simulink model "Final_Project"  (R2019a)
settings: Solver=VariableStepAuto  StartTime=0.0  StopTime=100.0  RelTol=1e-3
undefined symbols (not defined in the file): sigbuilder_block
libraries: nesl_utility x42, fl_lib x33, sh_lib x28
settings Model: Creator=danis  LastModifiedBy=danis

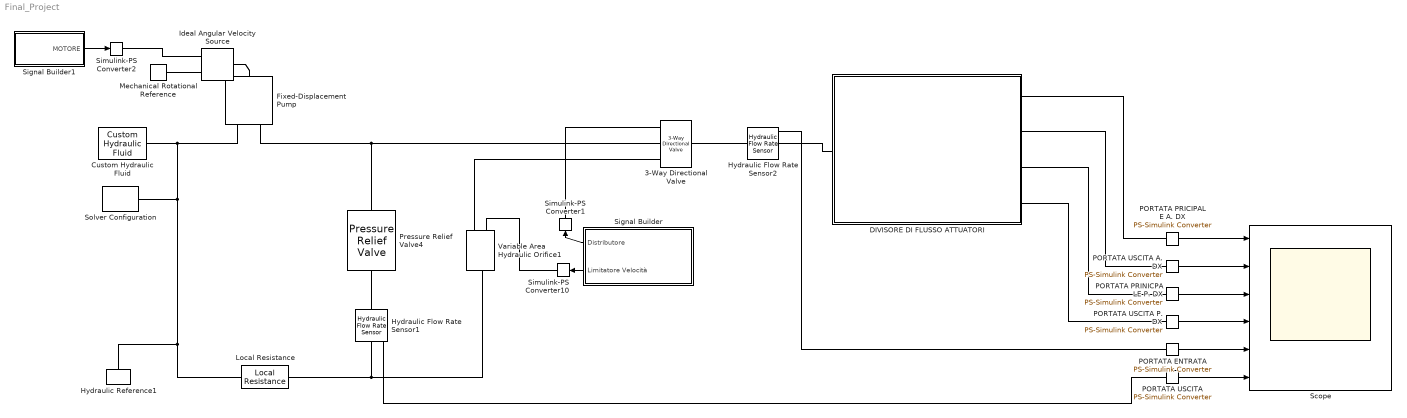
== system Final_Project ==
  3-Way Directional Valve : sh_lib/Valves/Directional Valves/3-Way Directional Valve  area_spec=sh.valves.directional_valves.enum.area_spec.identical  x_0_P=0 m  x_0_T=0 m  mdl_type_identical=sh.valves.directional_valves.enum.mdl_type.linear  mdl_type_different=sh.valves.directional_valves.enum.mdl_type.linear  opening_max=0.005 m  area_max=0.5e-4 m^2  opening_max_P_A=0.005 m  area_max_P_A=0.5e-4 m^2  opening_max_A_T=0.005 m  area_max_A_T=0.5e-4 m^2  opening_area_tab=[-.002, 0, .002, .005, .015] m  area_tab=[1e-09, 2.0352e-07, 4.0736e-05, .00011438, .00034356] m^2  opening_flow_rate_tab=[-.002, 0, .002, .005, .015] m  pressure_tab=[-10000000, -5000000, -2000000, 2000000, 5000000, 10000000] Pa  flow_rate_tab=[-1e-07, -7.0711e-08, -4.4721e-08, 4.4721e-08, 7.0711e-08, 1e-07; -2.0352e-05, -1.4391e-05, -9.1017e-06, 9.1017e-06, 1.4391e-05, 2.0352e-05; -.0040736, -.0028805, -.0018218, .0018218, .0028805, .0040736; -.011438, -.0080879, -.0051152, .0051152, .0080879, .011438; -.034356, -.024293, -.015364, .015364, .024293, .034356] m^3/s  opening_area_tab_P_A=[-.002, 0, .002, .005, .015] m  area_tab_P_A=[1e-09, 2.0352e-07, 4.0736e-05, .00011438, .00034356] m^2  opening_flow_rate_tab_P_A=[-.002, 0, .002, .005, .015] m  pressure_tab_P_A=[-10000000, -5000000, -2000000, 2000000, 5000000, 10000000] Pa  flow_rate_tab_P_A=[-1e-07, -7.0711e-08, -4.4721e-08, 4.4721e-08, 7.0711e-08, 1e-07; -2.0352e-05, -1.4391e-05, -9.1017e-06, 9.1017e-06, 1.4391e-05, 2.0352e-05; -.0040736, -.0028805, -.0018218, .0018218, .0028805, .0040736; -.011438, -.0080879, -.0051152, .0051152, .0080879, .011438; -.034356, -.024293, -.015364, .015364, .024293, .034356] m^3/s  opening_area_tab_A_T=[-.002, 0, .002, .005, .015] m  area_tab_A_T=[1e-09, 2.0352e-07, 4.0736e-05, .00011438, .00034356] m^2  opening_flow_rate_tab_A_T=[-.002, 0, .002, .005, .015] m  pressure_tab_A_T=[-10000000, -5000000, -2000000, 2000000, 5000000, 10000000] Pa  flow_rate_tab_A_T=[-1e-07, -7.0711e-08, -4.4721e-08, 4.4721e-08, 7.0711e-08, 1e-07; -2.0352e-05, -1.4391e-05, -9.1017e-06, 9.1017e-06, 1.4391e-05, 2.0352e-05; -.0040736, -.0028805, -.0018218, .0018218, .0028805, .0040736; -.011438, -.0080879, -.0051152, .0051152, .0080879, .011438; -.034356, -.024293, -.015364, .015364, .024293, .034356] m^3/s  interp_method_identical=sh.valves.directional_valves.enum.interp_method.linear  interp_method_different=sh.valves.directional_valves.enum.interp_method.linear  extrap_method_identical=sh.valves.directional_valves.enum.extrap_method.linear  extrap_method_different=sh.valves.directional_valves.enum.extrap_method.linear  A_leak=1e-15 m^2  C_d=0.7  lam_spec=sh.valves.directional_valves.enum.lam_spec.pressure_ratio  B_lam=0.999  Re_cr=12
      settings: SourceProductName=Simscape Fluids  SourceProductBaseCode=SH
  Custom Hydraulic Fluid : fl_lib/Hydraulic/Hydraulic Utilities/Custom Hydraulic Fluid  density=870 kg/m^3  viscosity_kin=0.000046 m^2/s  bulk=0.8e9 Pa  alpha=0.005  range_error=2
      settings: SourceProductName=Foundation Library
  DIVISORE DI FLUSSO ATTUATORI : Subsystem
  Fixed-Displacement Pump : sh_lib/Pumps and Motors/Fixed-Displacement Pump  D=10.5 cm^3/rev  loss_spec=1  w_nominal=952.4 rpm  pr_nominal=100e7 Pa  visc_nominal=0.000046 m^2/s  dens_nominal=870 kg/m^3  efficiency_vol=0.95  no_load_torque=0.0005 N*m  torque_pressure_coeff=0.6e-8 N*m/Pa  p_diff_eff_TLU=[100000, 1000000, 2000000] Pa  omega_eff_TLU=[25, 50, 100, 200, 300, 400] rad/s  vol_eff_TLU=[.816, .908, .954, .977, .981, .984; .325, .663, .831, .916, .925, .946; .137, .568, .78, .892, .893, .91]  mech_eff_TLU=[.996, .996, .996, .996, .996, .996; .988, .989, .989, .989, .989, .99; .981, .981, .982, .982, .983, .984]  p_diff_loss_TLU=[100000, 1000000, 2000000] Pa  omega_loss_TLU=[25, 50, 100, 200, 300, 400] rad/s  vol_loss_TLU=[.023, .023, .023, .023, .0285, .032; .0844, .0842, .0845, .084, .1125, .108; .1079, .108, .11, .108, .1605, .18] * 1e-3 m^3/s  mech_loss_TLU=[.002, .002, .002, .002, .002, .002; .0607, .0556, .0556, .0556, .0556, .0505; .1937, .1937, .1833, .1833, .1729, .1626] N*m  pressure_threshold=1e5 Pa  omega_threshold=10 rad/s  quadrant_check=0  pressure_check=0  min_valid_pressure=0 Pa  vol_eff_min=1e-3  vol_eff_max=1  mech_eff_min=1e-3  mech_eff_max=1
      settings: SourceProductName=Simscape Fluids  SourceProductBaseCode=SH
  Hydraulic Flow Rate Sensor1 : fl_lib/Hydraulic/Hydraulic Sensors/Hydraulic Flow Rate Sensor
      settings: SourceProductName=Simscape
  Hydraulic Flow Rate Sensor2 : fl_lib/Hydraulic/Hydraulic Sensors/Hydraulic Flow Rate Sensor
      settings: SourceProductName=Simscape
  Hydraulic Reference1 : fl_lib/Hydraulic/Hydraulic Elements/Hydraulic Reference
      settings: SourceProductName=Foundation Library
  Ideal Angular Velocity Source : fl_lib/Mechanical/Mechanical Sources/Ideal Angular Velocity Source
  Local Resistance : sh_lib/Local Hydraulic Resistances/Local Resistance  area=1e-4 m^2  mdl_type=1  kp_d=2  kp_r=2  lam_spec=1  B_lam=0.999  Re_cr=150  Re_vec=[-4000, -3000, -2000, -1000, -500, -200, -100, -50, -40, -30, -20, -15, -10, 10, 20, 30, 40, 50, 100, 200, 500, 1000, 2000, 4000, 5000, 10000]  loss_coeff_vec=[.25, .3, .65, .9, .65, .75, .9, 1.15, 1.35, 1.65, 2.3, 2.8, 3.1, 5, 2.7, 1.8, 1.46, 1.3, .9, .65, .42, .3, .2, .4, .42, .25]  interp_method=2  extrap_method=2  flow_rate_threshold=1e-6 m^3/s  flow_rate_specify=off  flow_rate_priority=None  flow_rate=0 m^3/s  flow_rate_nominal_specify=off  flow_rate_nominal_unit=m^3/s  flow_rate_nominal_value=1  pressure_drop_specify=off  pressure_drop_priority=None  pressure_drop=0 Pa  pressure_drop_nominal_specify=off  pressure_drop_nominal_unit=Pa  pressure_drop_nominal_value=1
      settings: SourceProductName=Simscape Fluids  SourceProductBaseCode=SH
  Mechanical Rotational Reference : fl_lib/Mechanical/Rotational Elements/Mechanical Rotational Reference
  PORTATA ENTRATA : nesl_utility/PS-Simulink Converter  PhysicalDomain=network_engine_domain  SubClassName=ps_output  LeftPortType=input  RightPortType=output  PseudoPeriodic=off  Frequencies=[]  Unit=1  AffineConversion=off
  PORTATA PRICIPALE A. DX : nesl_utility/PS-Simulink Converter  PhysicalDomain=network_engine_domain  SubClassName=ps_output  LeftPortType=input  RightPortType=output  PseudoPeriodic=off  Frequencies=[]  Unit=1  AffineConversion=off
  PORTATA PRINICPALE P. DX : nesl_utility/PS-Simulink Converter  PhysicalDomain=network_engine_domain  SubClassName=ps_output  LeftPortType=input  RightPortType=output  PseudoPeriodic=off  Frequencies=[]  Unit=1  AffineConversion=off
  "PORTATA USCITA " : nesl_utility/PS-Simulink Converter  PhysicalDomain=network_engine_domain  SubClassName=ps_output  LeftPortType=input  RightPortType=output  PseudoPeriodic=off  Frequencies=[]  Unit=1  AffineConversion=off
  PORTATA USCITA A. DX : nesl_utility/PS-Simulink Converter  PhysicalDomain=network_engine_domain  SubClassName=ps_output  LeftPortType=input  RightPortType=output  PseudoPeriodic=off  Frequencies=[]  Unit=1  AffineConversion=off
  PORTATA USCITA P. DX : nesl_utility/PS-Simulink Converter  PhysicalDomain=network_engine_domain  SubClassName=ps_output  LeftPortType=input  RightPortType=output  PseudoPeriodic=off  Frequencies=[]  Unit=1  AffineConversion=off
  Pressure Relief Valve4 : sh_lib/Valves/Pressure Control Valves/Pressure Relief Valve  valve_area_spec=1  p_diff_TLU=[30.15e5 : 15e3 : 31.35e5] Pa  area_TLU=[1 : 1 : 9] .* 1e-5 m^2  area_max=1e-4 m^2  pres_set=75 bar  reg_range=5 bar  C_d=0.7  A_leak=1e-15 m^2  lam_spec=1  B_lam=0.999  Re_cr=12  dynamic=0  tau=0.1 s  area_init=1e-12 m^2
      settings: SourceProductName=Simscape Fluids  SourceProductBaseCode=SH
  Scope : Scope  NumInputPorts=6
  Signal Builder : Subsystem  Tag=STV Subsys  LoadFcn=sigbuilder_block('load');  StartFcn=sigbuilder_block('start');  StopFcn=sigbuilder_block('stop');  ClipboardFcn=sigbuilder_block('clipboard');  mask(Sigbuilder block){tuvar=[0:10]}
      mask help: Simulink:masks:SigbuilderBlock_MD
      mask init:
      | if ~strcmp(get_param(bdroot(gcbh),'SimulationStatus'),'stopped') tuvar = sigbuilder_block('maskInit'); end
      settings: CopyFcn=sigbuilder_block('copy');  DeleteFcn=sigbuilder_block('delete');  ModelCloseFcn=sigbuilder_block('modelClose');  PreSaveFcn=sigbuilder_block('preSave');  PauseFcn=sigbuilder_block('pause');  ContinueFcn=sigbuilder_block('continue');  NameChangeFcn=sigbuilder_block('namechange');  OpenFcn=sigbuilder_block('open',[154.868 35.3208 673.811 360.679 ]);  CloseFcn=sigbuilder_block('close');
      mask Display: plot(0, 0, 100, 100,[2, 2, 32, 32, 2], [68, 8, 8, 68, 68],[32, 2], [38, 38], [32, 19, 2],[53, 60, 44], [32, 17, 17, 2],[16, 16, 31, 31]);txt = getActiveGroup(gcbh);text(2, 100, txt,'verticalAlignment', 'top');
  Signal Builder1 : Subsystem  Tag=STV Subsys  LoadFcn=sigbuilder_block('load');  StartFcn=sigbuilder_block('start');  StopFcn=sigbuilder_block('stop');  ClipboardFcn=sigbuilder_block('clipboard');  mask(Sigbuilder block){tuvar=[0:10]}
      mask help: Simulink:masks:SigbuilderBlock_MD
      mask init:
      | if ~strcmp(get_param(bdroot(gcbh),'SimulationStatus'),'stopped') tuvar = sigbuilder_block('maskInit'); end
      settings: CopyFcn=sigbuilder_block('copy');  DeleteFcn=sigbuilder_block('delete');  ModelCloseFcn=sigbuilder_block('modelClose');  PreSaveFcn=sigbuilder_block('preSave');  PauseFcn=sigbuilder_block('pause');  ContinueFcn=sigbuilder_block('continue');  NameChangeFcn=sigbuilder_block('namechange');  OpenFcn=sigbuilder_block('open',[371.547 99.1698 550.868 360.679 ]);  CloseFcn=sigbuilder_block('close');
      mask Display: plot(0, 0, 100, 100,[2, 2, 32, 32, 2], [68, 8, 8, 68, 68],[32, 2], [38, 38], [32, 19, 2],[53, 60, 44], [32, 17, 17, 2],[16, 16, 31, 31]);txt = getActiveGroup(gcbh);text(2, 100, txt,'verticalAlignment', 'top');
  Simulink-PS Converter1 : nesl_utility/Simulink-PS Converter  PhysicalDomain=network_engine_domain  SubClassName=ps_input  LeftPortType=input  RightPortType=output  PseudoPeriodic=off  Frequencies=[]  NoiseDistribution=none  NoiseParameters=[]  Unit=1  AffineConversion=off  FilteringAndDerivatives=provide  SimscapeFilterOrder=1  InputFilterTimeConstant=0.001  UdotUserProvided=0
  Simulink-PS Converter10 : nesl_utility/Simulink-PS Converter  PhysicalDomain=network_engine_domain  SubClassName=ps_input  LeftPortType=input  RightPortType=output  PseudoPeriodic=off  Frequencies=[]  NoiseDistribution=none  NoiseParameters=[]  Unit=1  AffineConversion=off  FilteringAndDerivatives=provide  SimscapeFilterOrder=1  InputFilterTimeConstant=0.001  UdotUserProvided=0
  Simulink-PS Converter2 : nesl_utility/Simulink-PS Converter  PhysicalDomain=network_engine_domain  SubClassName=ps_input  LeftPortType=input  RightPortType=output  PseudoPeriodic=off  Frequencies=[]  NoiseDistribution=none  NoiseParameters=[]  Unit=1  AffineConversion=off  FilteringAndDerivatives=provide  SimscapeFilterOrder=1  InputFilterTimeConstant=0.001  UdotUserProvided=0
  Solver Configuration : nesl_utility/Solver Configuration  PhysicalDomain=network_engine_domain  SubClassName=solver  LeftPortType=input  RightPortType=generic  Tones=[]  Harmonics=[]  SimulateNoise=off  Profile=off  UseLocalSampling=off  EnableSwitchedLinearOptims=on  FrequencyDomain=off  UseCCode=off  RelTol=0.001  AbsTol=1e-06  MinStep=1e-09  ToWorkspace=off  RevertToSquareIcSolve=off  NumHomotopyIterations=100  PhasorMode=off  PhasorModeNumHarmonics=1  DoDC=off  ResidualTolerance=1e-09  UseLocalSolver=off  LocalSolverChoice=NE_BACKWARD_EULER_ADVANCER  LocalSolverSampleTime=0.001  DoFixedCost=off  MaxNonlinIter=3  MaxModeIter=2  LinearAlgebra=auto  EquationFormulation=NE_TIME_EF  DelaysMemoryBudget=1024  AutomaticFiltering=on  FilteringTimeConstant=0.001  PartitionStorageMethod=AS_NEEDED  PartitionMemoryBudget=1024  PartitionMethod=FAST
  Variable Area Hydraulic Orifice1 : fl_lib/Hydraulic/Hydraulic Elements/Variable Area Hydraulic Orifice  C_d=0.7  min_area=1e-12 m^2  lam_spec=1  B_lam=0.999  Re_cr=12  q_specify=off  q_priority=None  q=0.001 m^3/s  q_nominal_specify=off  q_nominal_unit=m^3/s  q_nominal_value=1  p_specify=off  p_priority=None  p=0 Pa  p_nominal_specify=off  p_nominal_unit=Pa  p_nominal_value=1
      settings: SourceProductName=Simscape  SourceProductBaseCode=SS
  wires:
  Signal Builder/1(Distributore) -> Simulink-PS Converter1/1
  Signal Builder/2(Limitatore Velocità) -> Simulink-PS Converter10/1
  PORTATA PRICIPALE A. DX/1 -> Scope/1
  PORTATA USCITA A. DX/1 -> Scope/2
  PORTATA PRINICPALE P. DX/1 -> Scope/3
  PORTATA USCITA P. DX/1 -> Scope/4
  PORTATA ENTRATA/1 -> Scope/5
  "PORTATA USCITA "/1 -> Scope/6
  Signal Builder1/1(MOTORE) -> Simulink-PS Converter2/1
  connections:
  3-Way Directional Valve/RConn3 -- Variable Area Hydraulic Orifice1/LConn2
  Simulink-PS Converter10/RConn1 -- Variable Area Hydraulic Orifice1/LConn1
  Simulink-PS Converter1/RConn1 -- 3-Way Directional Valve/RConn1
  Hydraulic Flow Rate Sensor1/LConn1 -- Pressure Relief Valve4/RConn1
  Hydraulic Flow Rate Sensor2/RConn2 -- DIVISORE DI FLUSSO ATTUATORI/LConn1
  Hydraulic Reference1/LConn1 -- Fixed-Displacement Pump/RConn2 -- Custom Hydraulic Fluid/RConn1 -- Solver Configuration/RConn1 -- Local Resistance/RConn1
  Variable Area Hydraulic Orifice1/RConn1 -- Local Resistance/LConn1 -- Hydraulic Flow Rate Sensor1/RConn2
  3-Way Directional Valve/LConn1 -- Hydraulic Flow Rate Sensor2/LConn1
  DIVISORE DI FLUSSO ATTUATORI/RConn1 -- PORTATA PRICIPALE A. DX/LConn1
  DIVISORE DI FLUSSO ATTUATORI/RConn2 -- PORTATA USCITA A. DX/LConn1
  DIVISORE DI FLUSSO ATTUATORI/RConn3 -- PORTATA PRINICPALE P. DX/LConn1
  DIVISORE DI FLUSSO ATTUATORI/RConn4 -- PORTATA USCITA P. DX/LConn1
  Hydraulic Flow Rate Sensor2/RConn1 -- PORTATA ENTRATA/LConn1
  Hydraulic Flow Rate Sensor1/RConn1 -- "PORTATA USCITA "/LConn1
  Ideal Angular Velocity Source/LConn1 -- Fixed-Displacement Pump/LConn1
  Ideal Angular Velocity Source/RConn2 -- Mechanical Rotational Reference/LConn1
  Simulink-PS Converter2/RConn1 -- Ideal Angular Velocity Source/RConn1
  3-Way Directional Valve/RConn2 -- Fixed-Displacement Pump/RConn1 -- Pressure Relief Valve4/LConn1

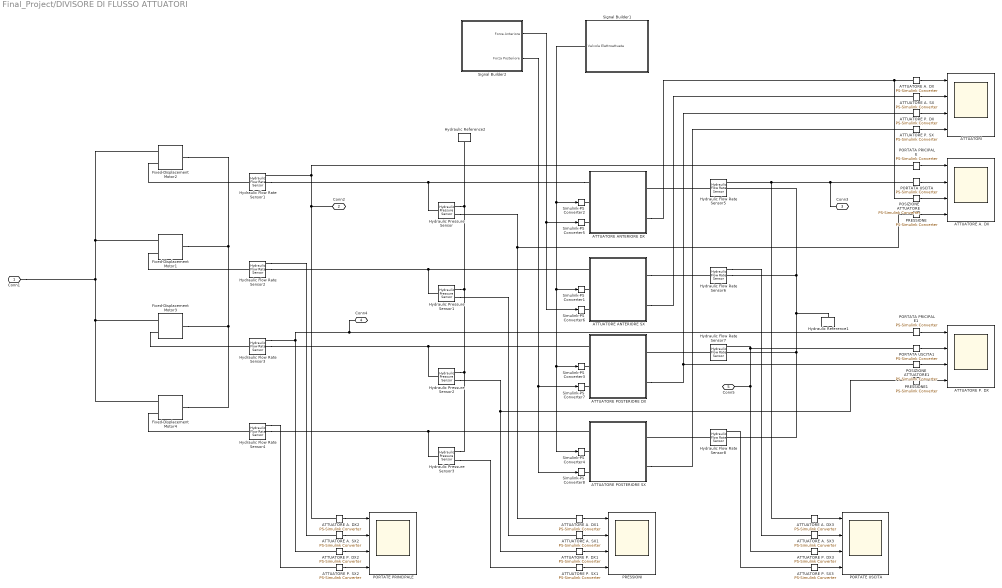
== system Final_Project/DIVISORE DI FLUSSO ATTUATORI ==
  ATTUATORE A. DX{,1..3} (4 alike) : nesl_utility/PS-Simulink Converter  PhysicalDomain=network_engine_domain  SubClassName=ps_output  LeftPortType=input  RightPortType=output  PseudoPeriodic=off  Frequencies=[]  Unit=1  AffineConversion=off
  "ATTUATORE A. DX " : Scope  NumInputPorts=4
  ATTUATORE A. SX{,1..3} (4 alike) : nesl_utility/PS-Simulink Converter  PhysicalDomain=network_engine_domain  SubClassName=ps_output  LeftPortType=input  RightPortType=output  PseudoPeriodic=off  Frequencies=[]  Unit=1  AffineConversion=off
  ATTUATORE ANTERIORE DX : Subsystem
  ATTUATORE ANTERIORE SX : Subsystem
  ATTUATORE P. DX{,1..3} (4 alike) : nesl_utility/PS-Simulink Converter  PhysicalDomain=network_engine_domain  SubClassName=ps_output  LeftPortType=input  RightPortType=output  PseudoPeriodic=off  Frequencies=[]  Unit=1  AffineConversion=off
  "ATTUATORE P. DX " : Scope  NumInputPorts=4
  ATTUATORE P. SX{,1..3} (4 alike) : nesl_utility/PS-Simulink Converter  PhysicalDomain=network_engine_domain  SubClassName=ps_output  LeftPortType=input  RightPortType=output  PseudoPeriodic=off  Frequencies=[]  Unit=1  AffineConversion=off
  ATTUATORE POSTERIORE DX : Subsystem
  ATTUATORE POSTERIORE SX : Subsystem
  ATTUATORI : Scope  NumInputPorts=4
  Fixed-Displacement Motor{1..4} (4 alike) : sh_lib/Pumps and Motors/Fixed-Displacement Motor  D=0.9 cm^3/rev  loss_spec=1  w_nominal=2777.8 rpm  pr_nominal=100e7 Pa  visc_nominal=0.000046 m^2/s  dens_nominal=870 kg/m^3  efficiency_vol=0.95  no_load_torque=0.0005 N*m  torque_pressure_coeff=0.6e-8 N*m/Pa  p_diff_eff_TLU=[100000, 1000000, 2000000] Pa  omega_eff_TLU=[25, 50, 100, 200, 300, 400] rad/s  vol_eff_TLU=[.816, .908, .954, .977, .981, .984; .325, .663, .831, .916, .925, .946; .137, .568, .78, .892, .893, .91]  mech_eff_TLU=[.996, .996, .996, .996, .996, .996; .988, .989, .989, .989, .989, .99; .981, .981, .982, .982, .983, .984]  p_diff_loss_TLU=[100000, 1000000, 2000000] Pa  omega_loss_TLU=[25, 50, 100, 200, 300, 400] rad/s  vol_loss_TLU=[.0282, .0253, .0241, .0235, .0291, .0325; .2596, .1271, .1017, .0917, .1216, .1142; .7874, .1901, .141, .1211, .1797, .1978] * 1e-3 m^3/s  mech_loss_TLU=[.002, .002, .002, .002, .002, .002; .06, .055, .055, .055, .055, .05; .19, .19, .18, .18, .17, .16] N*m  pressure_threshold=1e5 Pa  omega_threshold=10 rad/s  quadrant_check=0  pressure_check=0  min_valid_pressure=0 Pa  vol_eff_min=1e-3  vol_eff_max=1  mech_eff_min=1e-3  mech_eff_max=1
      settings: SourceProductName=Simscape Fluids  SourceProductBaseCode=SH
  Hydraulic Flow Rate Sensor{1..8} (8 alike) : fl_lib/Hydraulic/Hydraulic Sensors/Hydraulic Flow Rate Sensor
      settings: SourceProductName=Simscape
  Hydraulic Pressure Sensor{,1..3} (4 alike) : fl_lib/Hydraulic/Hydraulic Sensors/Hydraulic Pressure Sensor
      settings: SourceProductName=Simscape
  Hydraulic Reference1 : fl_lib/Hydraulic/Hydraulic Elements/Hydraulic Reference
      settings: SourceProductName=Foundation Library
  Hydraulic Reference2 : fl_lib/Hydraulic/Hydraulic Elements/Hydraulic Reference
      settings: SourceProductName=Foundation Library
  PORTATA PRICIPALE : nesl_utility/PS-Simulink Converter  PhysicalDomain=network_engine_domain  SubClassName=ps_output  LeftPortType=input  RightPortType=output  PseudoPeriodic=off  Frequencies=[]  Unit=1  AffineConversion=off
  PORTATA PRICIPALE1 : nesl_utility/PS-Simulink Converter  PhysicalDomain=network_engine_domain  SubClassName=ps_output  LeftPortType=input  RightPortType=output  PseudoPeriodic=off  Frequencies=[]  Unit=1  AffineConversion=off
  PORTATA USCITA : nesl_utility/PS-Simulink Converter  PhysicalDomain=network_engine_domain  SubClassName=ps_output  LeftPortType=input  RightPortType=output  PseudoPeriodic=off  Frequencies=[]  Unit=1  AffineConversion=off
  PORTATA USCITA1 : nesl_utility/PS-Simulink Converter  PhysicalDomain=network_engine_domain  SubClassName=ps_output  LeftPortType=input  RightPortType=output  PseudoPeriodic=off  Frequencies=[]  Unit=1  AffineConversion=off
  PORTATE PRINCIPALE : Scope  NumInputPorts=4
  PORTATE USCITA : Scope  NumInputPorts=4
  POSIZIONE ATTUATORE : nesl_utility/PS-Simulink Converter  PhysicalDomain=network_engine_domain  SubClassName=ps_output  LeftPortType=input  RightPortType=output  PseudoPeriodic=off  Frequencies=[]  Unit=1  AffineConversion=off
  POSIZIONE ATTUATORE1 : nesl_utility/PS-Simulink Converter  PhysicalDomain=network_engine_domain  SubClassName=ps_output  LeftPortType=input  RightPortType=output  PseudoPeriodic=off  Frequencies=[]  Unit=1  AffineConversion=off
  PRESSIONE : nesl_utility/PS-Simulink Converter  PhysicalDomain=network_engine_domain  SubClassName=ps_output  LeftPortType=input  RightPortType=output  PseudoPeriodic=off  Frequencies=[]  Unit=1  AffineConversion=off
  PRESSIONE1 : nesl_utility/PS-Simulink Converter  PhysicalDomain=network_engine_domain  SubClassName=ps_output  LeftPortType=input  RightPortType=output  PseudoPeriodic=off  Frequencies=[]  Unit=1  AffineConversion=off
  PRESSIONI : Scope  NumInputPorts=4
  Signal Builder1 : Subsystem  Tag=STV Subsys  LoadFcn=sigbuilder_block('load');  StartFcn=sigbuilder_block('start');  StopFcn=sigbuilder_block('stop');  ClipboardFcn=sigbuilder_block('clipboard');  mask(Sigbuilder block){tuvar=[0:10]}
      mask help: Simulink:masks:SigbuilderBlock_MD
      mask init:
      | if ~strcmp(get_param(bdroot(gcbh),'SimulationStatus'),'stopped') tuvar = sigbuilder_block('maskInit'); end
      settings: CopyFcn=sigbuilder_block('copy');  DeleteFcn=sigbuilder_block('delete');  ModelCloseFcn=sigbuilder_block('modelClose');  PreSaveFcn=sigbuilder_block('preSave');  PauseFcn=sigbuilder_block('pause');  ContinueFcn=sigbuilder_block('continue');  NameChangeFcn=sigbuilder_block('namechange');  OpenFcn=sigbuilder_block('open',[154.868 35.3208 673.811 360.679 ]);  CloseFcn=sigbuilder_block('close');
      mask Display: plot(0, 0, 100, 100,[2, 2, 32, 32, 2], [68, 8, 8, 68, 68],[32, 2], [38, 38], [32, 19, 2],[53, 60, 44], [32, 17, 17, 2],[16, 16, 31, 31]);txt = getActiveGroup(gcbh);text(2, 100, txt,'verticalAlignment', 'top');
  Signal Builder2 : Subsystem  Tag=STV Subsys  LoadFcn=sigbuilder_block('load');  StartFcn=sigbuilder_block('start');  StopFcn=sigbuilder_block('stop');  ClipboardFcn=sigbuilder_block('clipboard');  mask(Sigbuilder block){tuvar=[0:10]}
      mask help: Simulink:masks:SigbuilderBlock_MD
      mask init:
      | if ~strcmp(get_param(bdroot(gcbh),'SimulationStatus'),'stopped') tuvar = sigbuilder_block('maskInit'); end
      settings: CopyFcn=sigbuilder_block('copy');  DeleteFcn=sigbuilder_block('delete');  ModelCloseFcn=sigbuilder_block('modelClose');  PreSaveFcn=sigbuilder_block('preSave');  PauseFcn=sigbuilder_block('pause');  ContinueFcn=sigbuilder_block('continue');  NameChangeFcn=sigbuilder_block('namechange');  OpenFcn=sigbuilder_block('open',[146.717 99.1698 550.868 360.679 ]);  CloseFcn=sigbuilder_block('close');
      mask Display: plot(0, 0, 100, 100,[2, 2, 32, 32, 2], [68, 8, 8, 68, 68],[32, 2], [38, 38], [32, 19, 2],[53, 60, 44], [32, 17, 17, 2],[16, 16, 31, 31]);txt = getActiveGroup(gcbh);text(2, 100, txt,'verticalAlignment', 'top');
  Simulink-PS Converter{1..8} (8 alike) : nesl_utility/Simulink-PS Converter  PhysicalDomain=network_engine_domain  SubClassName=ps_input  LeftPortType=input  RightPortType=output  PseudoPeriodic=off  Frequencies=[]  NoiseDistribution=none  NoiseParameters=[]  Unit=1  AffineConversion=off  FilteringAndDerivatives=provide  SimscapeFilterOrder=1  InputFilterTimeConstant=0.001  UdotUserProvided=0
  Conn1 : PMIOPort  Side=Left
  Conn2 : PMIOPort  Port=2  Side=Right
  Conn3 : PMIOPort  Port=3  Side=Right
  Conn4 : PMIOPort  Port=4  Side=Right
  Conn5 : PMIOPort  Port=5  Side=Right
  wires:
  Signal Builder1/1(Valvola Elettroattuata) -> Simulink-PS Converter1/1, Simulink-PS Converter3/1, Simulink-PS Converter4/1, Simulink-PS Converter2/1
  Signal Builder2/1(Forza Anteriore) -> Simulink-PS Converter6/1, Simulink-PS Converter5/1
  Signal Builder2/2(Forza Posteriore) -> Simulink-PS Converter8/1, Simulink-PS Converter7/1
  ATTUATORE A. DX/1 -> ATTUATORI/1
  ATTUATORE A. SX/1 -> ATTUATORI/2
  ATTUATORE P. DX/1 -> ATTUATORI/3
  ATTUATORE P. SX/1 -> ATTUATORI/4
  ATTUATORE A. DX1/1 -> PRESSIONI/1
  ATTUATORE A. SX1/1 -> PRESSIONI/2
  ATTUATORE P. DX1/1 -> PRESSIONI/3
  ATTUATORE P. SX1/1 -> PRESSIONI/4
  ATTUATORE P. SX2/1 -> PORTATE PRINCIPALE/4
  ATTUATORE A. SX2/1 -> PORTATE PRINCIPALE/2
  ATTUATORE P. DX2/1 -> PORTATE PRINCIPALE/3
  ATTUATORE A. DX2/1 -> PORTATE PRINCIPALE/1
  ATTUATORE A. DX3/1 -> PORTATE USCITA/1
  ATTUATORE P. DX3/1 -> PORTATE USCITA/3
  ATTUATORE P. SX3/1 -> PORTATE USCITA/4
  ATTUATORE A. SX3/1 -> PORTATE USCITA/2
  PORTATA PRICIPALE/1 -> "ATTUATORE A. DX "/1
  POSIZIONE ATTUATORE/1 -> "ATTUATORE A. DX "/3
  PORTATA USCITA/1 -> "ATTUATORE A. DX "/2
  PRESSIONE/1 -> "ATTUATORE A. DX "/4
  PRESSIONE1/1 -> "ATTUATORE P. DX "/4
  PORTATA PRICIPALE1/1 -> "ATTUATORE P. DX "/1
  PORTATA USCITA1/1 -> "ATTUATORE P. DX "/2
  POSIZIONE ATTUATORE1/1 -> "ATTUATORE P. DX "/3
  connections:
  Fixed-Displacement Motor2/LConn1 -- Fixed-Displacement Motor1/LConn1 -- Conn1/RConn1 -- Fixed-Displacement Motor3/LConn1 -- Fixed-Displacement Motor4/LConn1
  Fixed-Displacement Motor2/RConn1 -- Fixed-Displacement Motor3/RConn1 -- Fixed-Displacement Motor4/RConn1 -- Fixed-Displacement Motor1/RConn1
  Hydraulic Flow Rate Sensor1/LConn1 -- Fixed-Displacement Motor2/LConn2
  Hydraulic Flow Rate Sensor2/RConn2 -- ATTUATORE ANTERIORE SX/LConn1 -- Hydraulic Pressure Sensor1/LConn1
  Hydraulic Flow Rate Sensor3/RConn2 -- ATTUATORE POSTERIORE DX/LConn1 -- Hydraulic Pressure Sensor2/LConn1
  Hydraulic Flow Rate Sensor5/RConn2 -- Hydraulic Reference1/LConn1 -- Hydraulic Flow Rate Sensor8/RConn2 -- Hydraulic Flow Rate Sensor7/RConn2 -- Hydraulic Flow Rate Sensor6/RConn2
  Hydraulic Flow Rate Sensor4/RConn2 -- ATTUATORE POSTERIORE SX/LConn1 -- Hydraulic Pressure Sensor3/LConn1
  Simulink-PS Converter2/RConn1 -- ATTUATORE ANTERIORE DX/LConn2
  Simulink-PS Converter1/RConn1 -- ATTUATORE ANTERIORE SX/LConn2
  Simulink-PS Converter3/RConn1 -- ATTUATORE POSTERIORE DX/LConn2
  Simulink-PS Converter4/RConn1 -- ATTUATORE POSTERIORE SX/LConn2
  Simulink-PS Converter5/RConn1 -- ATTUATORE ANTERIORE DX/LConn3
  Simulink-PS Converter6/RConn1 -- ATTUATORE ANTERIORE SX/LConn3
  Simulink-PS Converter7/RConn1 -- ATTUATORE POSTERIORE DX/LConn3
  Simulink-PS Converter8/RConn1 -- ATTUATORE POSTERIORE SX/LConn3
  ATTUATORE ANTERIORE DX/RConn2 -- POSIZIONE ATTUATORE/LConn1 -- ATTUATORE A. DX/LConn1
  ATTUATORE ANTERIORE SX/RConn2 -- ATTUATORE A. SX/LConn1
  ATTUATORE POSTERIORE DX/RConn2 -- POSIZIONE ATTUATORE1/LConn1 -- ATTUATORE P. DX/LConn1
  ATTUATORE POSTERIORE SX/RConn2 -- ATTUATORE P. SX/LConn1
  ATTUATORE ANTERIORE DX/LConn1 -- Hydraulic Flow Rate Sensor1/RConn2 -- Hydraulic Pressure Sensor/LConn1
  Fixed-Displacement Motor1/LConn2 -- Hydraulic Flow Rate Sensor2/LConn1
  Fixed-Displacement Motor3/LConn2 -- Hydraulic Flow Rate Sensor3/LConn1
  Fixed-Displacement Motor4/LConn2 -- Hydraulic Flow Rate Sensor4/LConn1
  Hydraulic Flow Rate Sensor5/LConn1 -- ATTUATORE ANTERIORE DX/RConn1
  ATTUATORE ANTERIORE SX/RConn1 -- Hydraulic Flow Rate Sensor6/LConn1
  Hydraulic Flow Rate Sensor7/LConn1 -- ATTUATORE POSTERIORE DX/RConn1
  Hydraulic Flow Rate Sensor8/LConn1 -- ATTUATORE POSTERIORE SX/RConn1
  Hydraulic Pressure Sensor/RConn1 -- Hydraulic Pressure Sensor3/RConn1 -- Hydraulic Pressure Sensor2/RConn1 -- Hydraulic Pressure Sensor1/RConn1 -- Hydraulic Reference2/LConn1
  Hydraulic Pressure Sensor/RConn2 -- PRESSIONE/LConn1 -- ATTUATORE A. DX1/LConn1
  Hydraulic Pressure Sensor1/RConn2 -- ATTUATORE A. SX1/LConn1
  Hydraulic Pressure Sensor2/RConn2 -- PRESSIONE1/LConn1 -- ATTUATORE P. DX1/LConn1
  Hydraulic Pressure Sensor3/RConn2 -- ATTUATORE P. SX1/LConn1
  Hydraulic Flow Rate Sensor3/RConn1 -- Conn4/RConn1 -- PORTATA PRICIPALE1/LConn1 -- ATTUATORE P. DX2/LConn1
  Hydraulic Flow Rate Sensor2/RConn1 -- ATTUATORE A. SX2/LConn1
  ATTUATORE P. SX3/LConn1 -- Hydraulic Flow Rate Sensor8/RConn1
  ATTUATORE P. DX3/LConn1 -- Conn5/RConn1 -- Hydraulic Flow Rate Sensor7/RConn1 -- PORTATA USCITA1/LConn1
  Hydraulic Flow Rate Sensor6/RConn1 -- ATTUATORE A. SX3/LConn1
  ATTUATORE A. DX3/LConn1 -- Conn3/RConn1 -- PORTATA USCITA/LConn1 -- Hydraulic Flow Rate Sensor5/RConn1
  Hydraulic Flow Rate Sensor4/RConn1 -- ATTUATORE P. SX2/LConn1
  ATTUATORE A. DX2/LConn1 -- PORTATA PRICIPALE/LConn1 -- Hydraulic Flow Rate Sensor1/RConn1 -- Conn2/RConn1

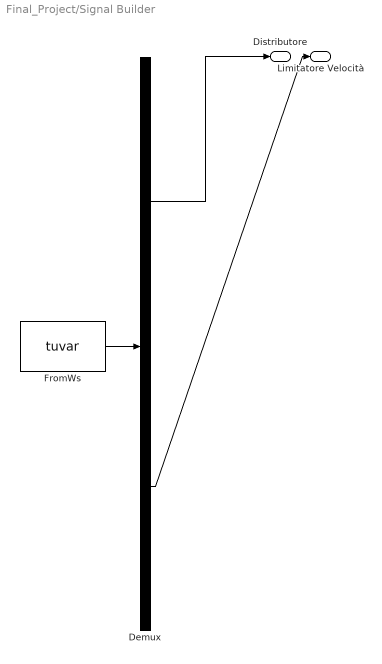
== system Final_Project/Signal Builder ==
  Demux : Demux  Tag=STV Demux  Outputs=2
  FromWs : FromWorkspace  Tag=STV FromWs  VariableName=tuvar  SampleTime=0
      SigBuilderData=|
      | common.afterFinalStr = 'Extrapolate'
      | common.sampleTime = 0
      | dataSet.timeRange = [0 100]
      | dataSet.name = 'Progetto'
      | sbobj.Groups.Name = 'Progetto'
      | sbobj.Groups.Signals(1).Name = 'Distributore'
      | sbobj.Groups.Signals(1).XData = [0 40 40 100]
      | sbobj.Groups.Signals(1).YData = [1 1 -1 -1]
      | sbobj.Groups.Signals(2).Name = 'Limitatore Velocità'
      | sbobj.Groups.Signals(2).XData = [0 100]
      | sbobj.Groups.Signals(2).YData = [2.3e-06 2.3e-06]
      | sbobj.Groups.TimeRange = [0 100]
  Distributore : Outport  Tag=STV Outport
  Limitatore Velocità : Outport  Tag=STV Outport  Port=2
  wires:
  Demux/1 -> Distributore/1
  FromWs/1 -> Demux/1
  Demux/2 -> Limitatore Velocità/1

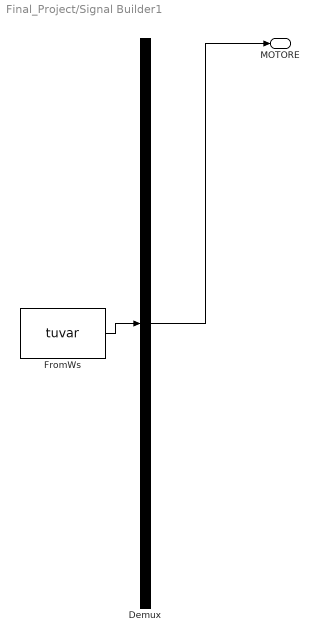
== system Final_Project/Signal Builder1 ==
  Demux : Demux  Tag=STV Demux  Outputs=1
  FromWs : FromWorkspace  Tag=STV FromWs  VariableName=tuvar  SampleTime=0
      SigBuilderData=|
      | common.afterFinalStr = 'Extrapolate'
      | common.sampleTime = 0
      | dataSet.timeRange = [0 100]
      | dataSet.name = 'Motore'
      | sbobj.Groups.Name = 'Motore'
      | sbobj.Groups.Signals.Name = 'MOTORE'
      | sbobj.Groups.Signals.XData = [0 100]
      | sbobj.Groups.Signals.YData = [100 100]
      | sbobj.Groups.TimeRange = [0 100]
  MOTORE : Outport  Tag=STV Outport
  wires:
  Demux/1 -> MOTORE/1
  FromWs/1 -> Demux/1

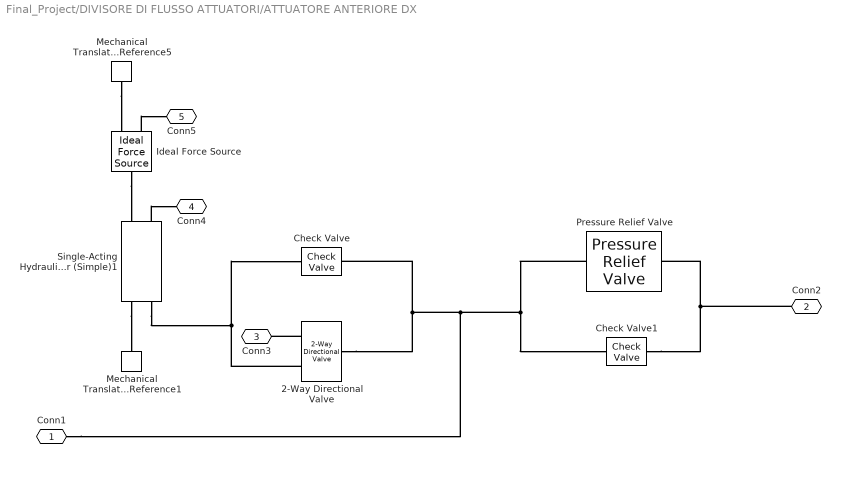
== system Final_Project/DIVISORE DI FLUSSO ATTUATORI/ATTUATORE ANTERIORE DX ==
  2-Way Directional Valve : sh_lib/Valves/Directional Valves/2-Way Directional Valve  mdl_type=1  area_max=0.5e-4 m^2  opening_max=0.005 m  opening_tab=[-.002, 0, .002, .005, .015] m  area_tab=[1e-09, 2.0352e-07, 4.0736e-05, .00011438, .00034356] m^2  pressure_tab=[-10000000, -5000000, -2000000, 2000000, 5000000, 10000000] Pa  flow_rate_tab=[-1e-07, -7.0711e-08, -4.4721e-08, 4.4721e-08, 7.0711e-08, 1e-07; -2.0352e-05, -1.4391e-05, -9.1017e-06, 9.1017e-06, 1.4391e-05, 2.0352e-05; -.0040736, -.0028805, -.0018218, .0018218, .0028805, .0040736; -.011438, -.0080879, -.0051152, .0051152, .0080879, .011438; -.034356, -.024293, -.015364, .015364, .024293, .034356] m^3/s  interp_method=1  extrap_method=1  C_d=0.7  x_0=0 m  A_leak=1e-15 m^2  lam_spec=1  B_lam=0.999  Re_cr=12
      settings: SourceProductName=Simscape Fluids  SourceProductBaseCode=SH
  Check Valve : sh_lib/Valves/Directional Valves/Check Valve  area_max=1e-4 m^2  pres_crack=1 bar  pres_max=2 bar  C_d=0.7  A_leak=1e-15 m^2  lam_spec=1  B_lam=0.999  Re_cr=12  dynamic=0  tau=0.1 s  area_init=1e-12 m^2
      settings: SourceProductName=Simscape Fluids  SourceProductBaseCode=SH
  Check Valve1 : sh_lib/Valves/Directional Valves/Check Valve  area_max=1e-4 m^2  pres_crack=0.1 bar  pres_max=1 bar  C_d=0.7  A_leak=1e-15 m^2  lam_spec=1  B_lam=0.999  Re_cr=12  dynamic=0  tau=0.1 s  area_init=1e-12 m^2
      settings: SourceProductName=Simscape Fluids  SourceProductBaseCode=SH
  Ideal Force Source : fl_lib/Mechanical/Mechanical Sources/Ideal Force Source
  Mechanical Translational Reference1 : fl_lib/Mechanical/Translational Elements/Mechanical Translational Reference
  Mechanical Translational Reference5 : fl_lib/Mechanical/Translational Elements/Mechanical Translational Reference
  Pressure Relief Valve : sh_lib/Valves/Pressure Control Valves/Pressure Relief Valve  valve_area_spec=1  p_diff_TLU=[30.15e5 : 15e3 : 31.35e5] Pa  area_TLU=[1 : 1 : 9] .* 1e-5 m^2  area_max=1e-4 m^2  pres_set=67.5 bar  reg_range=5 bar  C_d=0.7  A_leak=1e-15 m^2  lam_spec=1  B_lam=0.999  Re_cr=12  dynamic=0  tau=0.1 s  area_init=1e-12 m^2
      settings: SourceProductName=Simscape Fluids  SourceProductBaseCode=SH
  Single-Acting Hydraulic Cylinder (Simple)1 : sh_lib/Hydraulic Cylinders/Single-Acting Hydraulic Cylinder (Simple)  area=1.26e-3 m^2  stroke=1 m  init_pos=0 m  penetr_coeff=1e12 s*N/m^2  or=1
      settings: SourceProductName=Simscape Fluids  SourceProductBaseCode=SH
  Conn1 : PMIOPort  Side=Left
  Conn2 : PMIOPort  Port=2  Side=Right
  Conn3 : PMIOPort  Port=3  Side=Left
  Conn4 : PMIOPort  Port=4  Side=Right
  Conn5 : PMIOPort  Port=5  Side=Left
  connections:
  Single-Acting Hydraulic Cylinder (Simple)1/LConn1 -- Mechanical Translational Reference1/LConn1
  Pressure Relief Valve/LConn1 -- Conn1/RConn1 -- 2-Way Directional Valve/RConn1 -- Check Valve/LConn1 -- Check Valve1/RConn1
  Check Valve1/LConn1 -- Conn2/RConn1 -- Pressure Relief Valve/RConn1
  Ideal Force Source/RConn1 -- Conn5/RConn1
  Mechanical Translational Reference5/LConn1 -- Ideal Force Source/RConn2
  Ideal Force Source/LConn1 -- Single-Acting Hydraulic Cylinder (Simple)1/RConn1
  Single-Acting Hydraulic Cylinder (Simple)1/RConn2 -- Conn4/RConn1
  2-Way Directional Valve/LConn2 -- Check Valve/RConn1 -- Single-Acting Hydraulic Cylinder (Simple)1/LConn2
  2-Way Directional Valve/LConn1 -- Conn3/RConn1

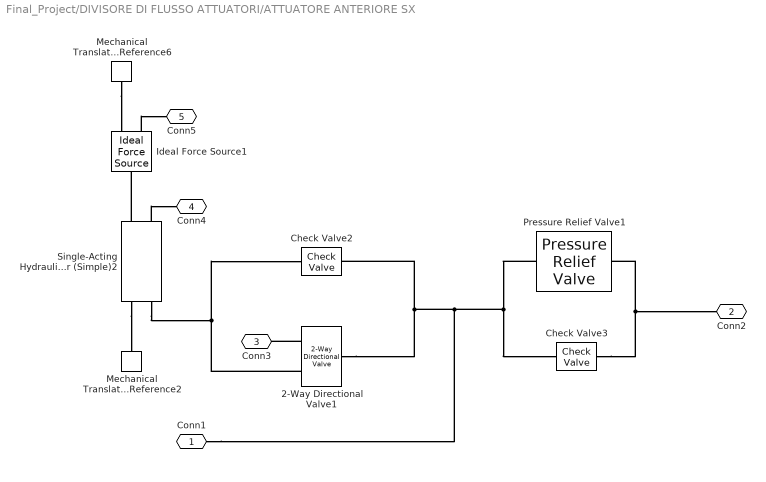
== system Final_Project/DIVISORE DI FLUSSO ATTUATORI/ATTUATORE ANTERIORE SX ==
  2-Way Directional Valve1 : sh_lib/Valves/Directional Valves/2-Way Directional Valve  mdl_type=1  area_max=0.5e-4 m^2  opening_max=0.005 m  opening_tab=[-.002, 0, .002, .005, .015] m  area_tab=[1e-09, 2.0352e-07, 4.0736e-05, .00011438, .00034356] m^2  pressure_tab=[-10000000, -5000000, -2000000, 2000000, 5000000, 10000000] Pa  flow_rate_tab=[-1e-07, -7.0711e-08, -4.4721e-08, 4.4721e-08, 7.0711e-08, 1e-07; -2.0352e-05, -1.4391e-05, -9.1017e-06, 9.1017e-06, 1.4391e-05, 2.0352e-05; -.0040736, -.0028805, -.0018218, .0018218, .0028805, .0040736; -.011438, -.0080879, -.0051152, .0051152, .0080879, .011438; -.034356, -.024293, -.015364, .015364, .024293, .034356] m^3/s  interp_method=1  extrap_method=1  C_d=0.7  x_0=0 m  A_leak=1e-15 m^2  lam_spec=1  B_lam=0.999  Re_cr=12
      settings: SourceProductName=Simscape Fluids  SourceProductBaseCode=SH
  Check Valve2 : sh_lib/Valves/Directional Valves/Check Valve  area_max=1e-4 m^2  pres_crack=1 bar  pres_max=2 bar  C_d=0.7  A_leak=1e-15 m^2  lam_spec=1  B_lam=0.999  Re_cr=12  dynamic=0  tau=0.1 s  area_init=1e-12 m^2
      settings: SourceProductName=Simscape Fluids  SourceProductBaseCode=SH
  Check Valve3 : sh_lib/Valves/Directional Valves/Check Valve  area_max=1e-4 m^2  pres_crack=0.1 bar  pres_max=1 bar  C_d=0.7  A_leak=1e-15 m^2  lam_spec=1  B_lam=0.999  Re_cr=12  dynamic=0  tau=0.1 s  area_init=1e-12 m^2
      settings: SourceProductName=Simscape Fluids  SourceProductBaseCode=SH
  Ideal Force Source1 : fl_lib/Mechanical/Mechanical Sources/Ideal Force Source
  Mechanical Translational Reference2 : fl_lib/Mechanical/Translational Elements/Mechanical Translational Reference
  Mechanical Translational Reference6 : fl_lib/Mechanical/Translational Elements/Mechanical Translational Reference
  Pressure Relief Valve1 : sh_lib/Valves/Pressure Control Valves/Pressure Relief Valve  valve_area_spec=1  p_diff_TLU=[30.15e5 : 15e3 : 31.35e5] Pa  area_TLU=[1 : 1 : 9] .* 1e-5 m^2  area_max=1e-4 m^2  pres_set=67.5 bar  reg_range=5 bar  C_d=0.7  A_leak=1e-15 m^2  lam_spec=1  B_lam=0.999  Re_cr=12  dynamic=0  tau=0.1 s  area_init=1e-12 m^2
      settings: SourceProductName=Simscape Fluids  SourceProductBaseCode=SH
  Single-Acting Hydraulic Cylinder (Simple)2 : sh_lib/Hydraulic Cylinders/Single-Acting Hydraulic Cylinder (Simple)  area=1.26e-3 m^2  stroke=1 m  init_pos=0 m  penetr_coeff=1e12 s*N/m^2  or=1
      settings: SourceProductName=Simscape Fluids  SourceProductBaseCode=SH
  Conn1 : PMIOPort  Side=Left
  Conn2 : PMIOPort  Port=2  Side=Right
  Conn3 : PMIOPort  Port=3  Side=Left
  Conn4 : PMIOPort  Port=4  Side=Right
  Conn5 : PMIOPort  Port=5  Side=Left
  connections:
  Ideal Force Source1/RConn1 -- Conn5/RConn1
  Pressure Relief Valve1/LConn1 -- Conn1/RConn1 -- Check Valve2/LConn1 -- 2-Way Directional Valve1/RConn1 -- Check Valve3/RConn1
  Check Valve3/LConn1 -- Pressure Relief Valve1/RConn1 -- Conn2/RConn1
  Mechanical Translational Reference6/LConn1 -- Ideal Force Source1/RConn2
  Single-Acting Hydraulic Cylinder (Simple)2/LConn1 -- Mechanical Translational Reference2/LConn1
  2-Way Directional Valve1/LConn2 -- Single-Acting Hydraulic Cylinder (Simple)2/LConn2 -- Check Valve2/RConn1
  Single-Acting Hydraulic Cylinder (Simple)2/RConn1 -- Ideal Force Source1/LConn1
  2-Way Directional Valve1/LConn1 -- Conn3/RConn1
  Single-Acting Hydraulic Cylinder (Simple)2/RConn2 -- Conn4/RConn1

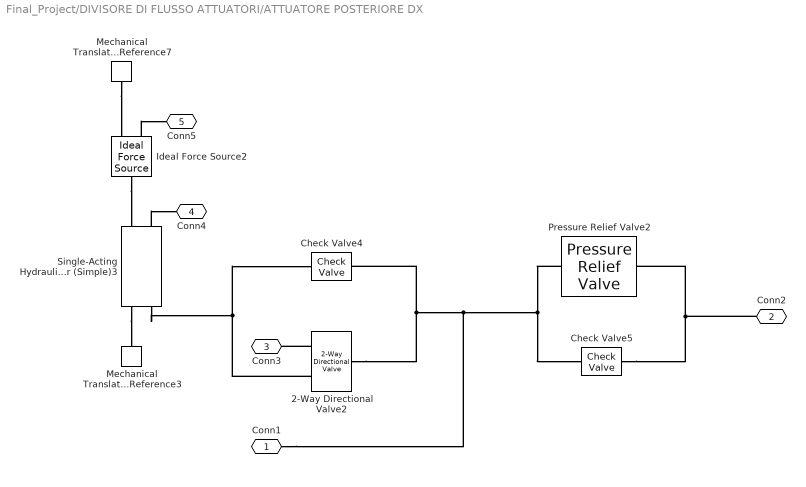
== system Final_Project/DIVISORE DI FLUSSO ATTUATORI/ATTUATORE POSTERIORE DX ==
  2-Way Directional Valve2 : sh_lib/Valves/Directional Valves/2-Way Directional Valve  mdl_type=1  area_max=0.5e-4 m^2  opening_max=0.005 m  opening_tab=[-.002, 0, .002, .005, .015] m  area_tab=[1e-09, 2.0352e-07, 4.0736e-05, .00011438, .00034356] m^2  pressure_tab=[-10000000, -5000000, -2000000, 2000000, 5000000, 10000000] Pa  flow_rate_tab=[-1e-07, -7.0711e-08, -4.4721e-08, 4.4721e-08, 7.0711e-08, 1e-07; -2.0352e-05, -1.4391e-05, -9.1017e-06, 9.1017e-06, 1.4391e-05, 2.0352e-05; -.0040736, -.0028805, -.0018218, .0018218, .0028805, .0040736; -.011438, -.0080879, -.0051152, .0051152, .0080879, .011438; -.034356, -.024293, -.015364, .015364, .024293, .034356] m^3/s  interp_method=1  extrap_method=1  C_d=0.7  x_0=0 m  A_leak=1e-15 m^2  lam_spec=1  B_lam=0.999  Re_cr=12
      settings: SourceProductName=Simscape Fluids  SourceProductBaseCode=SH
  Check Valve4 : sh_lib/Valves/Directional Valves/Check Valve  area_max=1e-4 m^2  pres_crack=1 bar  pres_max=2 bar  C_d=0.7  A_leak=1e-15 m^2  lam_spec=1  B_lam=0.999  Re_cr=12  dynamic=0  tau=0.1 s  area_init=1e-12 m^2
      settings: SourceProductName=Simscape Fluids  SourceProductBaseCode=SH
  Check Valve5 : sh_lib/Valves/Directional Valves/Check Valve  area_max=1e-4 m^2  pres_crack=0.1 bar  pres_max=1 bar  C_d=0.7  A_leak=1e-15 m^2  lam_spec=1  B_lam=0.999  Re_cr=12  dynamic=0  tau=0.1 s  area_init=1e-12 m^2
      settings: SourceProductName=Simscape Fluids  SourceProductBaseCode=SH
  Ideal Force Source2 : fl_lib/Mechanical/Mechanical Sources/Ideal Force Source
  Mechanical Translational Reference3 : fl_lib/Mechanical/Translational Elements/Mechanical Translational Reference
  Mechanical Translational Reference7 : fl_lib/Mechanical/Translational Elements/Mechanical Translational Reference
  Pressure Relief Valve2 : sh_lib/Valves/Pressure Control Valves/Pressure Relief Valve  valve_area_spec=1  p_diff_TLU=[30.15e5 : 15e3 : 31.35e5] Pa  area_TLU=[1 : 1 : 9] .* 1e-5 m^2  area_max=1e-4 m^2  pres_set=67.5 bar  reg_range=5 bar  C_d=0.7  A_leak=1e-15 m^2  lam_spec=1  B_lam=0.999  Re_cr=12  dynamic=0  tau=0.1 s  area_init=1e-12 m^2
      settings: SourceProductName=Simscape Fluids  SourceProductBaseCode=SH
  Single-Acting Hydraulic Cylinder (Simple)3 : sh_lib/Hydraulic Cylinders/Single-Acting Hydraulic Cylinder (Simple)  area=1.26e-3 m^2  stroke=1 m  init_pos=0 m  penetr_coeff=1e12 s*N/m^2  or=1
      settings: SourceProductName=Simscape Fluids  SourceProductBaseCode=SH
  Conn1 : PMIOPort  Side=Left
  Conn2 : PMIOPort  Port=2  Side=Right
  Conn3 : PMIOPort  Port=3  Side=Left
  Conn4 : PMIOPort  Port=4  Side=Right
  Conn5 : PMIOPort  Port=5  Side=Left
  connections:
  2-Way Directional Valve2/RConn1 -- Conn1/RConn1 -- Check Valve5/RConn1 -- Pressure Relief Valve2/LConn1 -- Check Valve4/LConn1
  Check Valve5/LConn1 -- Pressure Relief Valve2/RConn1 -- Conn2/RConn1
  Mechanical Translational Reference7/LConn1 -- Ideal Force Source2/RConn2
  Single-Acting Hydraulic Cylinder (Simple)3/LConn1 -- Mechanical Translational Reference3/LConn1
  Single-Acting Hydraulic Cylinder (Simple)3/RConn2 -- Conn4/RConn1
  Ideal Force Source2/RConn1 -- Conn5/RConn1
  2-Way Directional Valve2/LConn2 -- Single-Acting Hydraulic Cylinder (Simple)3/LConn2 -- Check Valve4/RConn1
  Ideal Force Source2/LConn1 -- Single-Acting Hydraulic Cylinder (Simple)3/RConn1
  2-Way Directional Valve2/LConn1 -- Conn3/RConn1

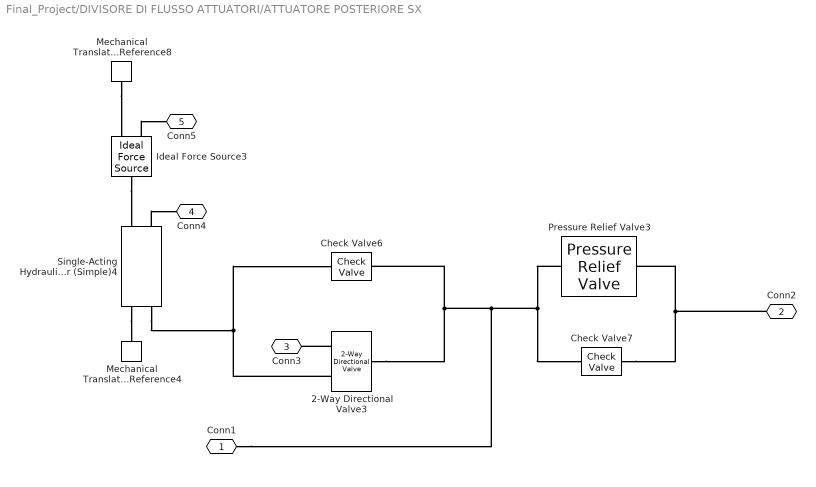
== system Final_Project/DIVISORE DI FLUSSO ATTUATORI/ATTUATORE POSTERIORE SX ==
  2-Way Directional Valve3 : sh_lib/Valves/Directional Valves/2-Way Directional Valve  mdl_type=1  area_max=0.5e-4 m^2  opening_max=0.005 m  opening_tab=[-.002, 0, .002, .005, .015] m  area_tab=[1e-09, 2.0352e-07, 4.0736e-05, .00011438, .00034356] m^2  pressure_tab=[-10000000, -5000000, -2000000, 2000000, 5000000, 10000000] Pa  flow_rate_tab=[-1e-07, -7.0711e-08, -4.4721e-08, 4.4721e-08, 7.0711e-08, 1e-07; -2.0352e-05, -1.4391e-05, -9.1017e-06, 9.1017e-06, 1.4391e-05, 2.0352e-05; -.0040736, -.0028805, -.0018218, .0018218, .0028805, .0040736; -.011438, -.0080879, -.0051152, .0051152, .0080879, .011438; -.034356, -.024293, -.015364, .015364, .024293, .034356] m^3/s  interp_method=1  extrap_method=1  C_d=0.7  x_0=0 m  A_leak=1e-15 m^2  lam_spec=1  B_lam=0.999  Re_cr=12
      settings: SourceProductName=Simscape Fluids  SourceProductBaseCode=SH
  Check Valve6 : sh_lib/Valves/Directional Valves/Check Valve  area_max=1e-4 m^2  pres_crack=1 bar  pres_max=2 bar  C_d=0.7  A_leak=1e-15 m^2  lam_spec=1  B_lam=0.999  Re_cr=12  dynamic=0  tau=0.1 s  area_init=1e-12 m^2
      settings: SourceProductName=Simscape Fluids  SourceProductBaseCode=SH
  Check Valve7 : sh_lib/Valves/Directional Valves/Check Valve  area_max=1e-4 m^2  pres_crack=0.1 bar  pres_max=1 bar  C_d=0.7  A_leak=1e-15 m^2  lam_spec=1  B_lam=0.999  Re_cr=12  dynamic=0  tau=0.1 s  area_init=1e-12 m^2
      settings: SourceProductName=Simscape Fluids  SourceProductBaseCode=SH
  Ideal Force Source3 : fl_lib/Mechanical/Mechanical Sources/Ideal Force Source
  Mechanical Translational Reference4 : fl_lib/Mechanical/Translational Elements/Mechanical Translational Reference
  Mechanical Translational Reference8 : fl_lib/Mechanical/Translational Elements/Mechanical Translational Reference
  Pressure Relief Valve3 : sh_lib/Valves/Pressure Control Valves/Pressure Relief Valve  valve_area_spec=1  p_diff_TLU=[30.15e5 : 15e3 : 31.35e5] Pa  area_TLU=[1 : 1 : 9] .* 1e-5 m^2  area_max=1e-4 m^2  pres_set=67.5 bar  reg_range=5 bar  C_d=0.7  A_leak=1e-15 m^2  lam_spec=1  B_lam=0.999  Re_cr=12  dynamic=0  tau=0.1 s  area_init=1e-12 m^2
      settings: SourceProductName=Simscape Fluids  SourceProductBaseCode=SH
  Single-Acting Hydraulic Cylinder (Simple)4 : sh_lib/Hydraulic Cylinders/Single-Acting Hydraulic Cylinder (Simple)  area=1.26e-3 m^2  stroke=1 m  init_pos=0 m  penetr_coeff=1e12 s*N/m^2  or=1
      settings: SourceProductName=Simscape Fluids  SourceProductBaseCode=SH
  Conn1 : PMIOPort  Side=Left
  Conn2 : PMIOPort  Port=2  Side=Right
  Conn3 : PMIOPort  Port=3  Side=Left
  Conn4 : PMIOPort  Port=4  Side=Right
  Conn5 : PMIOPort  Port=5  Side=Left
  connections:
  Pressure Relief Valve3/LConn1 -- Conn1/RConn1 -- 2-Way Directional Valve3/RConn1 -- Check Valve6/LConn1 -- Check Valve7/RConn1
  Ideal Force Source3/LConn1 -- Single-Acting Hydraulic Cylinder (Simple)4/RConn1
  Single-Acting Hydraulic Cylinder (Simple)4/RConn2 -- Conn4/RConn1
  2-Way Directional Valve3/LConn2 -- Check Valve6/RConn1 -- Single-Acting Hydraulic Cylinder (Simple)4/LConn2
  Mechanical Translational Reference8/LConn1 -- Ideal Force Source3/RConn2
  Check Valve7/LConn1 -- Pressure Relief Valve3/RConn1 -- Conn2/RConn1
  2-Way Directional Valve3/LConn1 -- Conn3/RConn1
  Single-Acting Hydraulic Cylinder (Simple)4/LConn1 -- Mechanical Translational Reference4/LConn1
  Ideal Force Source3/RConn1 -- Conn5/RConn1

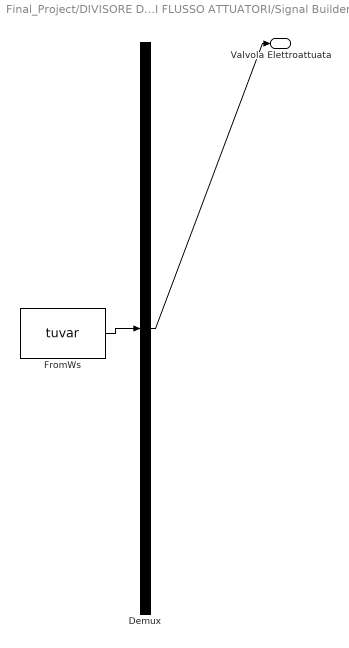
== system Final_Project/DIVISORE DI FLUSSO ATTUATORI/Signal Builder1 ==
  Demux : Demux  Tag=STV Demux  Outputs=1
  FromWs : FromWorkspace  Tag=STV FromWs  VariableName=tuvar  SampleTime=0
      SigBuilderData=|
      | common.afterFinalStr = 'Extrapolate'
      | common.sampleTime = 0
      | dataSet.timeRange = [0 100]
      | dataSet.name = 'CASSETTIERE'
      | sbobj.Groups.Name = 'CASSETTIERE'
      | sbobj.Groups.Signals.Name = 'Valvola Elettroattuata'
      | sbobj.Groups.Signals.XData = [0 50.2 50.2 100]
      | sbobj.Groups.Signals.YData = [-1 -1 0.98 0.98]
      | sbobj.Groups.TimeRange = [0 100]
  Valvola Elettroattuata : Outport  Tag=STV Outport
  wires:
  FromWs/1 -> Demux/1
  Demux/1 -> Valvola Elettroattuata/1

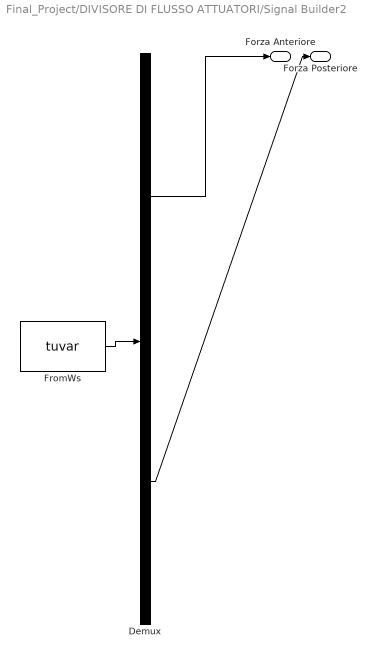
== system Final_Project/DIVISORE DI FLUSSO ATTUATORI/Signal Builder2 ==
  Demux : Demux  Tag=STV Demux  Outputs=2
  FromWs : FromWorkspace  Tag=STV FromWs  VariableName=tuvar  SampleTime=0
      SigBuilderData=|
      | common.afterFinalStr = 'Extrapolate'
      | common.sampleTime = 0
      | dataSet.timeRange = [0 100]
      | dataSet.name = 'FORZE'
      | sbobj.Groups.Name = 'FORZE'
      | sbobj.Groups.Signals(1).Name = 'Forza Anteriore'
      | sbobj.Groups.Signals(1).XData = [0 100]
      | sbobj.Groups.Signals(1).YData = [-7270 -7270]
      | sbobj.Groups.Signals(2).Name = 'Forza Posteriore'
      | sbobj.Groups.Signals(2).XData = [0 100]
      | sbobj.Groups.Signals(2).YData = [-5000 -5000]
      | sbobj.Groups.TimeRange = [0 100]
  Forza Anteriore : Outport  Tag=STV Outport
  Forza Posteriore : Outport  Tag=STV Outport  Port=2
  wires:
  Demux/1 -> Forza Anteriore/1
  FromWs/1 -> Demux/1
  Demux/2 -> Forza Posteriore/1
